simulink model "PreBrakingModel"  (Simulink 8.0)
settings: Solver=ode5  SolverMode=SingleTasking  StartTime=0.0  StopTime=inf  FixedStep=1/1000  RelTol=1e-3
libraries: simulink x27, simulink_extras x2
(part 1 of 2)
settings Model: Creator=Krzysztof  LastModifiedBy=battags  BufferReuse=off
settings DataIOCC: SignalLoggingSaveFormat=ModelDataLogs  SaveOutput=off  SaveTime=off
settings OptimizationCC: InlineParams=on  OptimizeBlockIOStorage=off  BufferReuse=off  ExpressionFolding=off  LocalBlockOutputs=off
settings DebuggingCC: SolverPrmCheckMsg=none  SigSpecEnsureSampleTimeMsg=none  ParameterPrecisionLossMsg=none  FcnCallInpInsideContextMsg=UseLocalSettings
settings ModelReferenceCC: ModelReferenceNumInstancesAllowed=Single
settings SFSimCC: SimParseCustomCode=off
settings GRTTargetCC: CombineOutputUpdateFcns=off  GRTInterface=on

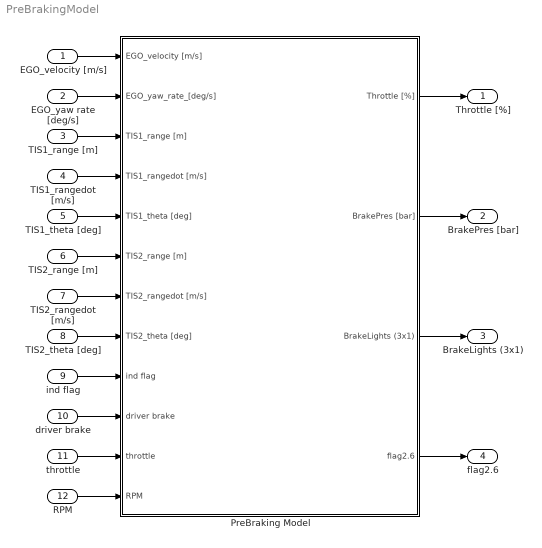
== system PreBrakingModel ==
  EGO_velocity [m/s] : Inport
  EGO_yaw rate [deg/s] : Inport  Port=2
  TIS1_range [m] : Inport  Port=3
  TIS1_rangedot [m/s] : Inport  Port=4
  TIS1_theta [deg] : Inport  Port=5
  TIS2_range [m] : Inport  Port=6
  TIS2_rangedot [m/s] : Inport  Port=7
  TIS2_theta [deg] : Inport  Port=8
  ind flag : Inport  Port=9
  driver brake : Inport  Port=10
  throttle : Inport  Port=11
  RPM : Inport  Port=12
  PreBraking Model : Subsystem  mask(PreBraking Model){MaxBrakePressure=150, BrakingPercent=0.4, LaneWidth=3.5, TISMaxRange=[150 30], TISMaxTheta=[9 80], Tblock=1/1000, Tsensor=[1/20 1/20], TISdet=[32 32], DisplaySwitch=off, DisplayFreq=20, RadarSwitch=off, RadarFreq=20}
      mask prompts: MaxBrakePressure "Maximum value of braking pressure [bar]"; BrakingPercent "Part of maximum braking pressure to use when partial braking [-]"; LaneWidth "Lane width [m]"; TISMaxRange "TIS maximum range (TIS1 and TIS2) [m]"; TISMaxTheta "TIS maximum theta angle (TIS1 and TIS2) [deg]"; Tblock "Target update rate of the compilation sheet [s]"; Tsensor "TIS update rate (TIS1 and TIS2) [s]"; TISdet "TIS max. objects to detect (TIS1 and TIS 2) [-]"; DisplaySwitch "Show EGO parameters visualization"; DisplayFreq "EGO parameters visualization frequency [Hz]"; RadarSwitch "Show radar visualization"; RadarFreq "Radar frequency [Hz]"
      mask help:
      | - intended to reduce speed of predicted collision,
      | - warns the driver and gives him more time to react,
      | - uses information from the state block
      |   and two independent TIS sensors,
      | - the system outputs are:
      |  = throttle and brake pressure (dynamics),
      |  = brake lights flags (light source visualisation animation)
      |  = the value of the warning flag.
      mask Callback DisplaySwitch:
      | en = get_param(gcb,'MaskEnables');
      | switch get_param(gcb, 'DisplaySwitch')
      |     case 'off'
      |         en{10} = 'off';
      |     case 'on'
      |         en{10} = 'on';
      | end
      | set_param(gcb,'MaskEnables',en);
      mask Callback RadarSwitch:
      | en = get_param(gcb,'MaskEnables');
      | switch get_param(gcb, 'RadarSwitch')
      |     case 'off'
      |         en{12} = 'off';
      |     case 'on'
      |         en{12} = 'on';
      | end
      | set_param(gcb,'MaskEnables',en);
  Throttle [%] : Outport
  BrakePres [bar] : Outport  Port=2
  BrakeLights (3x1) : Outport  Port=3
  flag2.6 : Outport  Port=4
  wires:
  PreBraking Model/1(Throttle [%]) -> Throttle [%]/1
  PreBraking Model/2(BrakePres [bar]) -> BrakePres [bar]/1
  PreBraking Model/3(BrakeLights (3x1)) -> BrakeLights (3x1)/1
  PreBraking Model/4(flag2.6) -> flag2.6/1
  EGO_velocity [m/s]/1 -> PreBraking Model/1(EGO_velocity [m/s])
  TIS1_range [m]/1 -> PreBraking Model/3(TIS1_range [m])
  TIS1_rangedot [m/s]/1 -> PreBraking Model/4(TIS1_rangedot [m/s])
  TIS1_theta [deg]/1 -> PreBraking Model/5(TIS1_theta [deg])
  TIS2_range [m]/1 -> PreBraking Model/6(TIS2_range [m])
  TIS2_rangedot [m/s]/1 -> PreBraking Model/7(TIS2_rangedot [m/s])
  TIS2_theta [deg]/1 -> PreBraking Model/8(TIS2_theta [deg])
  ind flag/1 -> PreBraking Model/9(ind flag)
  driver brake/1 -> PreBraking Model/10(driver brake)
  throttle/1 -> PreBraking Model/11(throttle)
  EGO_yaw rate [deg/s]/1 -> PreBraking Model/2(EGO_yaw_rate_[deg/s])
  RPM/1 -> PreBraking Model/12(RPM)

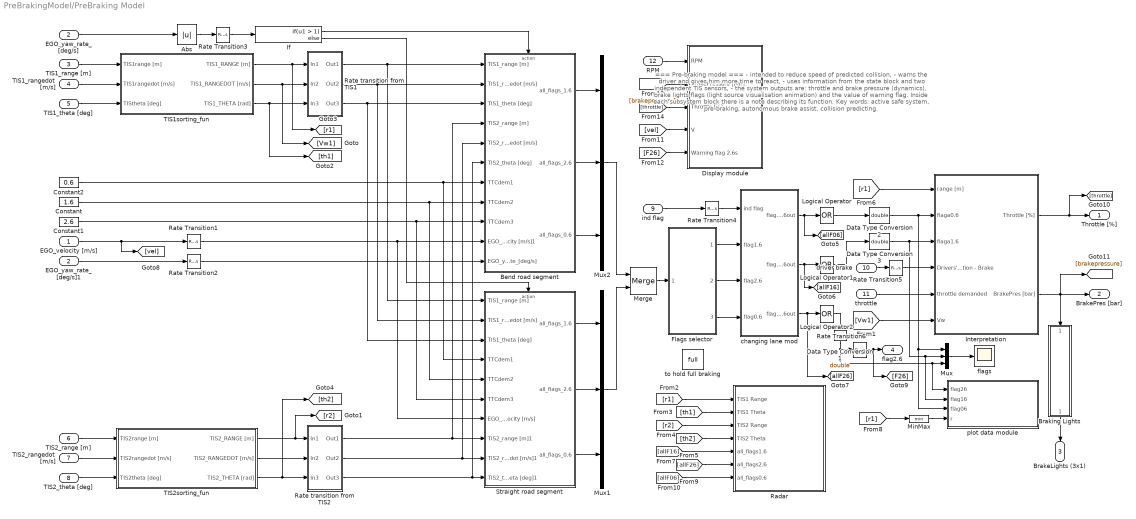
== system PreBrakingModel/PreBraking Model ==
  note: === Pre-braking model ===
      |
      |    - intended to reduce speed of predicted collision,
      |    - warns the driver and gives him more time to react,
      |    - uses information from the state block and two independent TIS sensors,
      |    - the system outputs are: throttle and brake pressure (dynamics),
      |      brake lights flags (light source visualisation animation) and the value of warning flag.
      |
      |    Inside each subsystem block there is a note describing its function.
      |
      |    Key words:
      |       active safe system, pre-braking, autonomous brake assist, collision predicting.
  EGO_velocity [m/s] : Inport  SampleTime=Tblock
  EGO_yaw_rate_[deg/s] : Inport  Port=2  SampleTime=Tblock
  TIS1_range [m] : Inport  Port=3  PortDimensions=TISdet(1)  SampleTime=Tsensor(1)
  TIS1_rangedot [m/s] : Inport  Port=4  PortDimensions=TISdet(1)  SampleTime=Tsensor(1)
  TIS1_theta [deg] : Inport  Port=5  PortDimensions=TISdet(1)  SampleTime=Tsensor(1)
  TIS2_range [m] : Inport  Port=6  PortDimensions=TISdet(2)  SampleTime=Tsensor(2)
  TIS2_rangedot [m/s] : Inport  Port=7  PortDimensions=TISdet(2)  SampleTime=Tsensor(2)
  TIS2_theta [deg] : Inport  Port=8  PortDimensions=TISdet(2)  SampleTime=Tsensor(2)
  ind flag : Inport  Port=9  SampleTime=[0 0]
  driver brake : Inport  Port=10  SampleTime=[0 0]
  throttle : Inport  Port=11  SampleTime=[0 0]
  RPM : Inport  Port=12  SampleTime=Tblock
  Abs : Abs
  Bend road segment : Subsystem  TreatAsAtomicUnit=on
  Braking Lights : Subsystem
  Constant : Constant  Value=1.6
  Constant1 : Constant  Value=2.6
  Constant2 : Constant  Value=0.6
  Data Type Conversion1 : DataTypeConversion  OutDataTypeStr=double
  Data Type Conversion2 : DataTypeConversion  OutDataTypeStr=double
  Data Type Conversion3 : DataTypeConversion  OutDataTypeStr=double
  Display module : Subsystem
  EGO_yaw_rate_[deg/s]1 : InportShadow  Port=2  SampleTime=Tblock
  Flags selector : Subsystem
  If : If  IfExpression=u1 > 1  SampleTime=min(Tsensor)
  Interpretation : Subsystem
  Logical Operator : Logic  Operator=OR  Inputs=1  AllPortsSameDT=off  OutDataTypeStr=boolean
  Logical Operator1 : Logic  Operator=OR  Inputs=1  AllPortsSameDT=off  OutDataTypeStr=boolean
  Logical Operator2 : Logic  Operator=OR  Inputs=1  AllPortsSameDT=off  OutDataTypeStr=boolean
  Merge : Merge
  MinMax : MinMax
  Mux : Mux  Inputs=3
  Mux1 : Mux  Inputs=3
  Mux2 : Mux  Inputs=3
  Radar : Subsystem
  Rate Transition{1..5} (5 alike) : RateTransition  Integrity=off  OutPortSampleTime=min(Tsensor)
  Rate Transition6 : RateTransition  Integrity=off  OutPortSampleTime=0
  Rate transition from TIS1 : Subsystem
  Rate transition from TIS2 : Subsystem
  Straight road segment : Subsystem  TreatAsAtomicUnit=on
  TIS1sorting_fun : Subsystem
  TIS2sorting_fun : Subsystem
  changing lane mod : Subsystem
  flags : Scope
      settings: TimeRange=0.1284900331530992  YMin=0.9893455251653903  YMax=1  SaveName=ScopeData26
  plot data module : Subsystem
  to hold full braking : DataStoreMemory  DataStoreName=full
  Throttle [%] : Outport
  BrakePres [bar] : Outport  Port=2
  BrakeLights (3x1) : Outport  Port=3
  flag2.6 : Outport  Port=4
  wires:
  Braking Lights/1(BrakeLights (3x1)) -> BrakeLights (3x1)/1
  driver brake/1 -> Rate Transition5/1
  throttle/1 -> Interpretation/5(throttle demanded)
  ind flag/1 -> Rate Transition4/1
  MinMax/1 -> plot data module/4(r)
  Mux/1 -> flags/1
  [r1] -> Interpretation/1(range [m])
  [r1] -> MinMax/1
  changing lane mod/1(flag0.6out) -> Logical Operator/1, [allF06]
  changing lane mod/2(flag1.6out) -> Logical Operator1/1, [allF16]
  changing lane mod/3(flag2.6out) -> Logical Operator2/1, [allF26]
  Interpretation/1(Throttle [%]) -> Throttle [%]/1, [throttle]
  If/2 -> Straight road segment/Action
  If/1 -> Bend road segment/Action
  Interpretation/2(BrakePres [bar]) -> Braking Lights/1(BrakePres), BrakePres [bar]/1, [brakepressure]
  Abs/1 -> Rate Transition3/1
  [Vw1] -> Interpretation/6(Vw)
  TIS1sorting_fun/1(TIS1_RANGE [m]) -> Rate transition from TIS1/1(In1), [r1]
  TIS1sorting_fun/2(TIS1_RANGEDOT [m/s]) -> [Vw1], Rate transition from TIS1/2(In2)
  Constant2/1 -> Bend road segment/7(TTCdem1), Straight road segment/4(TTCdem1)
  Constant/1 -> Bend road segment/8(TTCdem2), Straight road segment/5(TTCdem2)
  Constant1/1 -> Bend road segment/9(TTCdem3), Straight road segment/6(TTCdem3)
  EGO_velocity [m/s]/1 -> Rate Transition1/1, [vel]
  Mux2/1 -> Merge/1
  Mux1/1 -> Merge/2
  EGO_yaw_rate_[deg/s]1/1 -> Rate Transition2/1
  EGO_yaw_rate_[deg/s]/1 -> Abs/1
  TIS1_range [m]/1 -> TIS1sorting_fun/1(TIS1range [m])
  TIS1_rangedot [m/s]/1 -> TIS1sorting_fun/2(TIS1rangedot [m/s])
  TIS1_theta [deg]/1 -> TIS1sorting_fun/3(TIStheta [deg])
  TIS2_range [m]/1 -> TIS2sorting_fun/1(TIS2range [m])
  TIS2_rangedot [m/s]/1 -> TIS2sorting_fun/2(TIS2rangedot [m/s])
  TIS2_theta [deg]/1 -> TIS2sorting_fun/3(TIS2theta [deg])
  TIS1sorting_fun/3(TIS1_THETA [rad]) -> Rate transition from TIS1/3(In3), [th1]
  Rate transition from TIS1/1(Out1) -> Straight road segment/1(TIS1_range [m]), Bend road segment/1(TIS1_range [m])
  Rate transition from TIS1/2(Out2) -> Bend road segment/2(TIS1_rangedot [m/s]), Straight road segment/2(TIS1_rangedot [m/s])
  Rate transition from TIS1/3(Out3) -> Straight road segment/3(TIS1_theta [deg]), Bend road segment/3(TIS1_theta [deg])
  TIS2sorting_fun/1(TIS2_RANGE [m]) -> Rate transition from TIS2/1(In1), [r2]
  TIS2sorting_fun/2(TIS2_RANGEDOT [m/s]) -> Rate transition from TIS2/2(In2)
  TIS2sorting_fun/3(TIS2_THETA [rad]) -> Rate transition from TIS2/3(In3), [th2]
  Rate transition from TIS2/1(Out1) -> Straight road segment/8(TIS2_range [m]1), Bend road segment/4(TIS2_range [m])
  Rate transition from TIS2/2(Out2) -> Straight road segment/9(TIS2_rangedot [m/s]1), Bend road segment/5(TIS2_rangedot [m/s])
  Rate transition from TIS2/3(Out3) -> Straight road segment/10(TIS2_theta [deg]1), Bend road segment/6(TIS2_theta [deg])
  Rate Transition1/1 -> Bend road segment/10(EGO_velocity [m/s]1), Straight road segment/7(EGO_velocity [m/s])
  Rate Transition2/1 -> Bend road segment/11(EGO_yaw_rate_[deg/s])
  Rate Transition4/1 -> changing lane mod/1(ind flag)
  Rate Transition3/1 -> If/1
  Rate Transition5/1 -> Interpretation/4(Drivers's Reaction - Brake)
  Rate Transition6/1 -> flag2.6/1, [F26]
  Bend road segment/1(all_flags_1.6) -> Mux2/1
  Bend road segment/2(all_flags_2.6) -> Mux2/2
  Bend road segment/3(all_flags_0.6) -> Mux2/3
  Straight road segment/1(all_flags_1.6) -> Mux1/1
  Straight road segment/2(all_flags_2.6) -> Mux1/2
  Straight road segment/3(all_flags_0.6) -> Mux1/3
  Merge/1 -> Flags selector/1(all_flags)
  [r1] -> Radar/1(TIS1 Range)
  [th1] -> Radar/2(TIS1 Theta)
  [r2] -> Radar/3(TIS2 Range)
  [th2] -> Radar/4(TIS2 Theta)
  [allF16] -> Radar/5(all_flags1.6)
  [allF26] -> Radar/6(all_flags2.6)
  [allF06] -> Radar/7(all_flags0.6)
  [vel] -> Display module/4(V)
  [F26] -> Display module/5(Warning flag 2.6s)
  RPM/1 -> Display module/1(RPM)
  [brakepressure] -> Display module/2(BrakePressure [bar])
  [throttle] -> Display module/3(Throttle [%])
  Flags selector/1(all_flags1.6) -> changing lane mod/2(flag1.6)
  Flags selector/2(all_flags2.6) -> changing lane mod/3(flag2.6)
  Flags selector/3(all_flags0.6) -> changing lane mod/4(flag0.6)
  Logical Operator/1 -> Data Type Conversion2/1
  Logical Operator1/1 -> Data Type Conversion3/1
  Logical Operator2/1 -> Data Type Conversion1/1
  Data Type Conversion1/1 -> Mux/3, plot data module/1(flag26), Rate Transition6/1
  Data Type Conversion2/1 -> Mux/1, plot data module/3(flag06), Interpretation/2(flaga0.6)
  Data Type Conversion3/1 -> Interpretation/3(flaga1.6), Mux/2, plot data module/2(flag16)

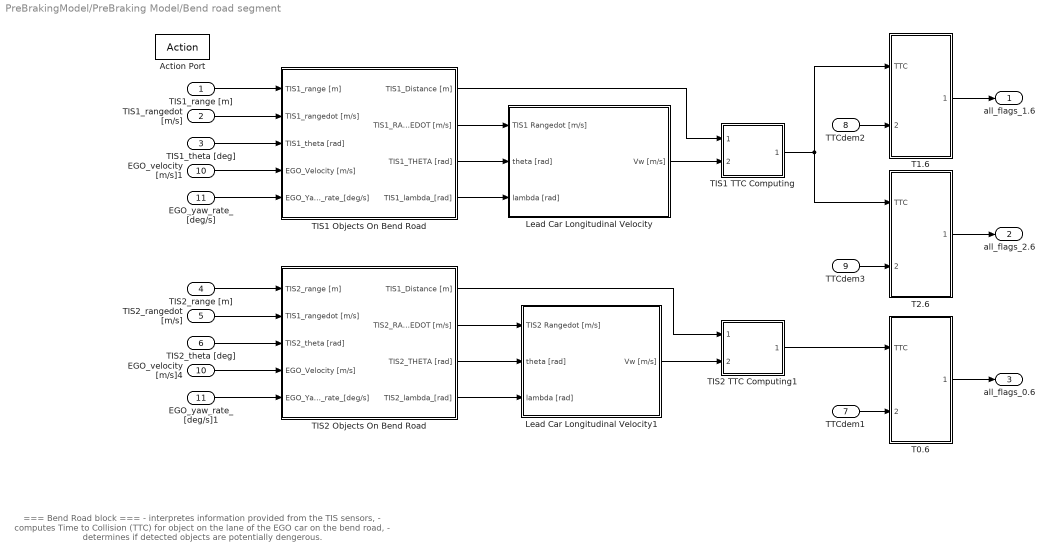
== system PreBrakingModel/PreBraking Model/Bend road segment ==
  note: === Bend Road block ===
      |
      |  - interpretes information provided from the TIS sensors,
      |  - computes Time to Collision (TTC) for object on the lane of the EGO car on the bend road,
      |  - determines if detected objects are potentially dengerous.
  TIS1_range [m] : Inport  PortDimensions=TISdet(1)
  TIS1_rangedot [m/s] : Inport  Port=2  PortDimensions=TISdet(1)
  TIS1_theta [deg] : Inport  Port=3  PortDimensions=TISdet(1)
  TIS2_range [m] : Inport  Port=4  PortDimensions=TISdet(2)
  TIS2_rangedot [m/s] : Inport  Port=5  PortDimensions=TISdet(2)
  TIS2_theta [deg] : Inport  Port=6  PortDimensions=TISdet(2)
  TTCdem1 : Inport  Port=7
  TTCdem2 : Inport  Port=8
  TTCdem3 : Inport  Port=9
  EGO_velocity [m/s]1 : Inport  Port=10
  EGO_yaw_rate_[deg/s] : Inport  Port=11
  Action Port : ActionPort  PropagateVarSize=During execution  ActionType=then
  EGO_velocity [m/s]4 : InportShadow  Port=10
  EGO_yaw_rate_[deg/s]1 : InportShadow  Port=11
  Lead Car Longitudinal Velocity : Subsystem
  Lead Car Longitudinal Velocity1 : Subsystem
  T0.6 : Subsystem
  T1.6 : Subsystem
  T2.6 : Subsystem
  TIS1 Objects On Bend Road : Subsystem
  TIS1 TTC Computing : Subsystem
  TIS2 Objects On Bend Road : Subsystem
  TIS2 TTC Computing1 : Subsystem
  all_flags_1.6 : Outport
  all_flags_2.6 : Outport  Port=2
  all_flags_0.6 : Outport  Port=3
  wires:
  EGO_yaw_rate_[deg/s]/1 -> TIS1 Objects On Bend Road/5(EGO_Yaw_rate_[deg/s])
  EGO_yaw_rate_[deg/s]1/1 -> TIS2 Objects On Bend Road/5(EGO_Yaw_rate_[deg/s])
  Lead Car Longitudinal Velocity1/1(Vw [m/s]) -> TIS2 TTC Computing1/2(Velocity [m/s])
  EGO_velocity [m/s]1/1 -> TIS1 Objects On Bend Road/4(EGO_Velocity [m/s])
  EGO_velocity [m/s]4/1 -> TIS2 Objects On Bend Road/4(EGO_Velocity [m/s])
  TIS1 Objects On Bend Road/2(TIS1_RANGEDOT [m/s]) -> Lead Car Longitudinal Velocity/1(TIS1 Rangedot [m/s])
  TIS1 Objects On Bend Road/3(TIS1_THETA [rad]) -> Lead Car Longitudinal Velocity/2(theta [rad])
  TIS1 Objects On Bend Road/4(TIS1_lambda_[rad]) -> Lead Car Longitudinal Velocity/3(lambda [rad])
  TIS2 Objects On Bend Road/1(TIS1_Distance [m]) -> TIS2 TTC Computing1/1(Distance [m])
  TIS2 Objects On Bend Road/2(TIS2_RANGEDOT [m/s]) -> Lead Car Longitudinal Velocity1/1(TIS2 Rangedot [m/s])
  TIS2 Objects On Bend Road/3(TIS2_THETA [rad]) -> Lead Car Longitudinal Velocity1/2(theta [rad])
  TIS2 Objects On Bend Road/4(TIS2_lambda_[rad]) -> Lead Car Longitudinal Velocity1/3(lambda [rad])
  TIS1 Objects On Bend Road/1(TIS1_Distance [m]) -> TIS1 TTC Computing/1(Distance [m])
  Lead Car Longitudinal Velocity/1(Vw [m/s]) -> TIS1 TTC Computing/2(Velocity [m/s])
  TIS1_range [m]/1 -> TIS1 Objects On Bend Road/1(TIS1_range [m])
  TIS1_rangedot [m/s]/1 -> TIS1 Objects On Bend Road/2(TIS1_rangedot [m/s])
  TIS1_theta [deg]/1 -> TIS1 Objects On Bend Road/3(TIS1_theta [rad])
  TIS2_range [m]/1 -> TIS2 Objects On Bend Road/1(TIS2_range [m])
  TIS2_rangedot [m/s]/1 -> TIS2 Objects On Bend Road/2(TIS1_rangedot [m/s])
  TIS2_theta [deg]/1 -> TIS2 Objects On Bend Road/3(TIS2_theta [rad])
  TTCdem2/1 -> T1.6/2(Constant TTC)
  TIS1 TTC Computing/1(TTC [s]) -> T1.6/1(TTC), T2.6/1(TTC)
  TTCdem3/1 -> T2.6/2(Constant TTC)
  TIS2 TTC Computing1/1(TTC [s]) -> T0.6/1(TTC)
  TTCdem1/1 -> T0.6/2(Constant TTC)
  T1.6/1(all_flags_1.6) -> all_flags_1.6/1
  T2.6/1(all_flags_2.6) -> all_flags_2.6/1
  T0.6/1(all_flags_0.6) -> all_flags_0.6/1

== system PreBrakingModel/PreBraking Model/Braking Lights ==
  note: === Braking lights block ===
      |
      |    - according to brake pressure, lights up braking lights of the actor,
      |    - the signal is a 3x1 vector:
      |      = first        value - left braking light,
      |      = second value - middle braking light,
      |      = third       value - right braking light.
  BrakePres : Inport
  Compare : simulink/Logic and Bit Operations/Compare To Constant  relop===  const=MaxBrakePressure  OutDataTypeStr=uint8
  Constant : Constant
  Constant1 : Constant  Value=0
  If : If  ShowElse=off  SampleTime=Tblock
  If Action Subsystem : Subsystem  TreatAsAtomicUnit=on
  Mux : Mux  Inputs=3
  Pulse Generator : DiscretePulseGenerator  Period=60  PulseWidth=30  SampleTime=Tblock
  Rate Transition2 : RateTransition  OutPortSampleTime=Tblock
  Switch : Switch  Criteria=u2 ~= 0
  Switch1 : Switch  Threshold=MaxBrakePressure
  Switch2 : Switch  Threshold=MaxBrakePressure
  BrakeLights (3x1) : Outport
  wires:
  Mux/1 -> BrakeLights (3x1)/1
  BrakePres/1 -> Rate Transition2/1
  Constant/1 -> Switch/1
  Switch/1 -> Mux/2, Switch1/3, Switch2/3
  Constant1/1 -> Switch/3
  Compare/1 -> If/1
  If/1 -> If Action Subsystem/Action
  Pulse Generator/1 -> If Action Subsystem/1(In1)
  If Action Subsystem/1(left light) -> Switch2/1
  If Action Subsystem/2(right light) -> Switch1/1
  Switch2/1 -> Mux/1
  Switch1/1 -> Mux/3
  Rate Transition2/1 -> Compare/1, Switch/2, Switch1/2, Switch2/2

== system PreBrakingModel/PreBraking Model/Display module ==
  RPM : Inport
  BrakePressure [bar] : Inport  Port=2
  Throttle [%] : Inport  Port=3
  V : Inport  Port=4
  Warning flag 2.6s : Inport  Port=5
  Display : Subsystem
  Display switch : Constant  Value=DisplaySwitch  SampleTime=1/DisplayFreq
  Gain : Gain  Gain=3.6
  Rate Transition{,1..4} (5 alike) : RateTransition  Integrity=off  OutPortSampleTime=1/DisplayFreq
  wires:
  BrakePressure [bar]/1 -> Rate Transition3/1
  Throttle [%]/1 -> Rate Transition4/1
  Warning flag 2.6s/1 -> Rate Transition/1
  RPM/1 -> Rate Transition1/1
  V/1 -> Gain/1
  Rate Transition1/1 -> Display/1(RPM)
  Rate Transition2/1 -> Display/2(V)
  Rate Transition3/1 -> Display/3(BrakePressure)
  Rate Transition4/1 -> Display/4(Throttle)
  Rate Transition/1 -> Display/5(Warning flag 2.6s)
  Display switch/1 -> Display/Enable
  Gain/1 -> Rate Transition2/1

== system PreBrakingModel/PreBraking Model/Flags selector ==
  all_flags : Inport
  Constant : Constant  Value=0
  Constant1 : Constant
  Data Store Read1 : DataStoreRead  DataStoreName=full  SampleTime=min(Tsensor)
  Data Type Conversion : DataTypeConversion
  Gain : Gain  Gain=ones(TISdet(1),1)
  Gain1 : Gain  Gain=ones(TISdet(1),1)
  Logical Operator : Logic  Operator=OR  Inputs=1  AllPortsSameDT=off  OutDataTypeStr=boolean
  Selector : Selector  InputPortWidth=2*TISdet(1)+TISdet(2)  IndexOptions=Starting index (dialog)  Indices=1  OutputSizes=TISdet(1)
  Selector1 : Selector  InputPortWidth=2*TISdet(1)+TISdet(2)  IndexOptions=Starting index (dialog)  Indices=TISdet(1)+1  OutputSizes=TISdet(1)
  Selector2 : Selector  InputPortWidth=2*TISdet(1)+TISdet(2)  IndexOptions=Starting index (dialog)  Indices=2* TISdet(1)+1  OutputSizes=TISdet(2)
  Sum : Sum  Inputs=++++
  Switch1 : Switch  Criteria=u2 > Threshold
  all_flags1.6 : Outport
  all_flags2.6 : Outport  Port=2
  all_flags0.6 : Outport  Port=3
  wires:
  Selector/1 -> all_flags1.6/1, Sum/1
  Selector2/1 -> all_flags0.6/1, Logical Operator/1
  all_flags/1 -> Data Type Conversion/1
  Data Type Conversion/1 -> Selector1/1, Selector/1, Selector2/1
  Selector1/1 -> Sum/2
  Data Store Read1/1 -> Gain/1
  Gain/1 -> Sum/4
  Logical Operator/1 -> Gain1/1
  Gain1/1 -> Sum/3
  Sum/1 -> Switch1/2
  Constant1/1 -> Switch1/1
  Constant/1 -> Switch1/3
  Switch1/1 -> all_flags2.6/1

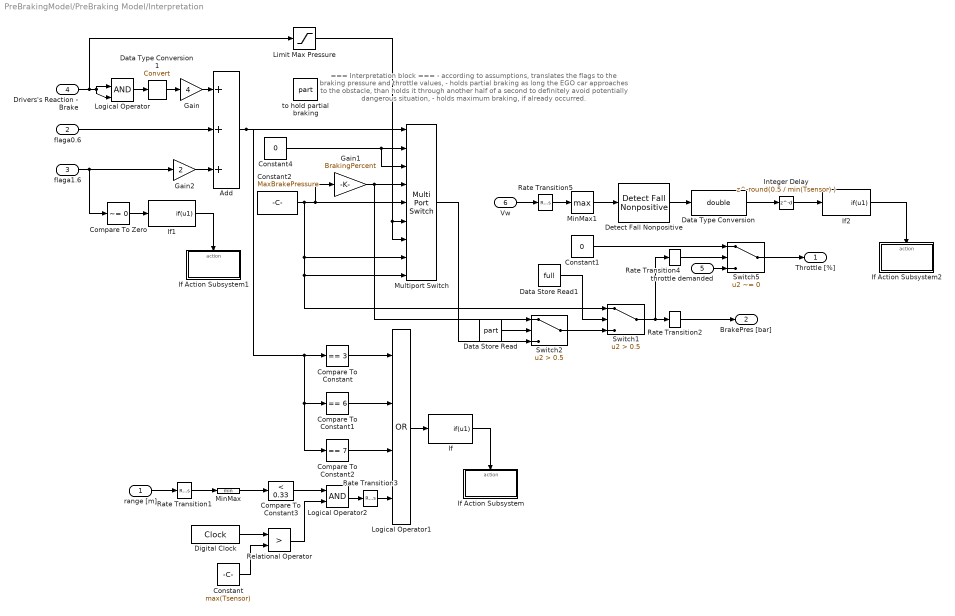
== system PreBrakingModel/PreBraking Model/Interpretation ==
  note: === Interpretation block ===
      |
      |    - according to assumptions, translates the flags
      |      to the braking pressure and throttle values,
      |    - holds partial braking as long the EGO car
      |      approaches to the obstacle, than holds it
      |      through another half of a second to definitely
      |      avoid potentially dangerous situation,
      |    - holds maximum braking, if already occurred.
  range [m] : Inport
  flaga0.6 : Inport  Port=2
  flaga1.6 : Inport  Port=3
  Drivers's Reaction - Brake : Inport  Port=4
  throttle demanded : Inport  Port=5  SampleTime=0
  Vw : Inport  Port=6
  Add : Sum  Inputs=3  SampleTime=min(Tsensor)
  Compare To Constant : simulink/Logic and Bit Operations/Compare To Constant  relop===  const=3  OutDataTypeStr=uint8
  Compare To Constant1 : simulink/Logic and Bit Operations/Compare To Constant  relop===  const=6  OutDataTypeStr=uint8
  Compare To Constant2 : simulink/Logic and Bit Operations/Compare To Constant  relop===  const=7  OutDataTypeStr=uint8
  Compare To Constant3 : simulink/Logic and Bit Operations/Compare To Constant  relop=<  const=0.33  OutDataTypeStr=uint8
  Compare To Zero : simulink/Logic and Bit Operations/Compare To Zero  relop=~=  OutDataTypeStr=uint8
  Constant : Constant  Value=max(Tsensor)
  Constant1 : Constant  Value=0  SampleTime=0
  Constant2 : Constant  Value=MaxBrakePressure  OutDataTypeStr=double  SampleTime=min(Tsensor)
  Constant4 : Constant  Value=0  SampleTime=min(Tsensor)
  Data Store Read : DataStoreRead  DataStoreName=part  SampleTime=min(Tsensor)
  Data Store Read1 : DataStoreRead  DataStoreName=full  SampleTime=min(Tsensor)
  Data Type Conversion : DataTypeConversion  OutDataTypeStr=double
  Data Type Conversion1 : DataTypeConversion
  Detect Fall Nonpositive : simulink/Logic and Bit Operations/Detect Fall Nonpositive  vinit=0  InputProcessing=Inherited  OutDataTypeStr=uint8
  Digital Clock : DigitalClock  SampleTime=min(Tsensor)
  Gain : Gain  Gain=4  SampleTime=min(Tsensor)
  Gain1 : Gain  Gain=BrakingPercent
  Gain2 : Gain  Gain=2
  If : If  IfExpression=u1  ShowElse=off  SampleTime=min(Tsensor)
  If Action Subsystem : Subsystem  TreatAsAtomicUnit=on
  If Action Subsystem1 : Subsystem  TreatAsAtomicUnit=on
  If Action Subsystem2 : Subsystem  TreatAsAtomicUnit=on
  If1 : If  IfExpression=u1  ShowElse=off
  If2 : If  IfExpression=u1  ShowElse=off  SampleTime=min(Tsensor)
  Integer Delay : Delay  DelayLength=round(0.5 / min(Tsensor) )  InputProcessing=Inherited
  Limit Max Pressure : Saturate  UpperLimit=MaxBrakePressure  LowerLimit=0  SampleTime=min(Tsensor)
  Logical Operator : Logic  IconShape=distinctive  AllPortsSameDT=off  OutDataTypeStr=boolean  SampleTime=min(Tsensor)
  Logical Operator1 : Logic  Operator=OR  Inputs=4  AllPortsSameDT=off  OutDataTypeStr=boolean  SampleTime=min(Tsensor)
  Logical Operator2 : Logic  AllPortsSameDT=off  OutDataTypeStr=boolean
  MinMax : MinMax
  MinMax1 : MinMax  Function=max
  Multiport Switch : MultiPortSwitch  DataPortOrder=Zero-based contiguous  Inputs=8  zeroidx=on
  Rate Transition1 : RateTransition  Integrity=off  OutPortSampleTime=min(Tsensor)
  Rate Transition2 : RateTransition  Integrity=off  OutPortSampleTime=0
  Rate Transition3 : RateTransition  Integrity=off  OutPortSampleTime=min(Tsensor)
  Rate Transition4 : RateTransition  Integrity=off  OutPortSampleTime=0
  Rate Transition5 : RateTransition  Integrity=off  OutPortSampleTime=min(Tsensor)
  Relational Operator : RelationalOperator  Operator=>  OutDataTypeStr=boolean  SampleTime=min(Tsensor)
  Switch1 : Switch  Criteria=u2 > Threshold  Threshold=0.5  SampleTime=min(Tsensor)
  Switch2 : Switch  Criteria=u2 > Threshold  Threshold=0.5  SampleTime=min(Tsensor)
  Switch5 : Switch  Criteria=u2 ~= 0
  to hold partial braking : DataStoreMemory  DataStoreName=part
  Throttle [%] : Outport  SampleTime=0
  BrakePres [bar] : Outport  Port=2
  wires:
  flaga1.6/1 -> Gain2/1, Compare To Zero/1
  Drivers's Reaction - Brake/1 -> Logical Operator/1, Logical Operator/2, Limit Max Pressure/1
  Gain2/1 -> Add/3
  Add/1 -> Multiport Switch/1, Compare To Constant1/1, Compare To Constant2/1, Compare To Constant/1
  Constant2/1 -> Gain1/1, Multiport Switch/5, Multiport Switch/8, Multiport Switch/9, Switch1/1
  flaga0.6/1 -> Add/2
  Gain/1 -> Add/1
  Multiport Switch/1 -> Switch2/3
  throttle demanded/1 -> Switch5/3
  Logical Operator/1 -> Data Type Conversion1/1
  Constant4/1 -> Multiport Switch/2, Multiport Switch/3
  Gain1/1 -> Multiport Switch/4, Switch2/1
  Limit Max Pressure/1 -> Multiport Switch/6, Multiport Switch/7
  range [m]/1 -> Rate Transition1/1
  Compare To Constant/1 -> Logical Operator1/1
  Compare To Constant1/1 -> Logical Operator1/2
  Compare To Constant2/1 -> Logical Operator1/3
  Logical Operator1/1 -> If/1
  Data Store Read/1 -> Switch2/2
  If/1 -> If Action Subsystem/Action
  MinMax/1 -> Compare To Constant3/1
  If1/1 -> If Action Subsystem1/Action
  Data Store Read1/1 -> Switch1/2
  Switch2/1 -> Switch1/3
  Compare To Zero/1 -> If1/1
  Vw/1 -> Rate Transition5/1
  MinMax1/1 -> Detect Fall Nonpositive/1
  If2/1 -> If Action Subsystem2/Action
  Detect Fall Nonpositive/1 -> Data Type Conversion/1
  Data Type Conversion/1 -> Integer Delay/1
  Integer Delay/1 -> If2/1
  Switch5/1 -> Throttle [%]/1
  Switch1/1 -> Rate Transition4/1, Rate Transition2/1
  Constant1/1 -> Switch5/1
  Rate Transition1/1 -> MinMax/1
  Digital Clock/1 -> Relational Operator/1
  Logical Operator2/1 -> Rate Transition3/1
  Compare To Constant3/1 -> Logical Operator2/1
  Relational Operator/1 -> Logical Operator2/2
  Rate Transition3/1 -> Logical Operator1/4
  Constant/1 -> Relational Operator/2
  Rate Transition5/1 -> MinMax1/1
  Rate Transition4/1 -> Switch5/2
  Rate Transition2/1 -> BrakePres [bar]/1
  Data Type Conversion1/1 -> Gain/1

== system PreBrakingModel/PreBraking Model/Radar ==
  TIS1 Range : Inport
  TIS1 Theta : Inport  Port=2
  TIS2 Range : Inport  Port=3
  TIS2 Theta : Inport  Port=4
  all_flags1.6 : Inport  Port=5
  all_flags2.6 : Inport  Port=6
  all_flags0.6 : Inport  Port=7
  Radar : Subsystem
  Radar switch : Constant  Value=RadarSwitch
  Rate Transition{1..7} (7 alike) : RateTransition  Integrity=off  OutPortSampleTime=1/RadarFreq
  wires:
  TIS1 Range/1 -> Rate Transition5/1
  TIS1 Theta/1 -> Rate Transition1/1
  TIS2 Range/1 -> Rate Transition2/1
  TIS2 Theta/1 -> Rate Transition3/1
  all_flags1.6/1 -> Rate Transition4/1
  all_flags2.6/1 -> Rate Transition6/1
  all_flags0.6/1 -> Rate Transition7/1
  Rate Transition5/1 -> Radar/1(TIS1 Range)
  Rate Transition1/1 -> Radar/2(TIS1 Theta)
  Rate Transition2/1 -> Radar/3(TIS2 Range)
  Rate Transition3/1 -> Radar/4(TIS2 Theta)
  Rate Transition4/1 -> Radar/5(all_flags1.6)
  Rate Transition6/1 -> Radar/6(all_flags2.6)
  Rate Transition7/1 -> Radar/7(all_flags0.6)
  Radar switch/1 -> Radar/Enable

== system PreBrakingModel/PreBraking Model/Rate transition from TIS1 ==
  In1 : Inport
  In2 : Inport  Port=2
  In3 : Inport  Port=3
  Rate Transition1 : RateTransition  Integrity=off  OutPortSampleTime=min(Tsensor)
  Rate Transition2 : RateTransition  Integrity=off  OutPortSampleTime=min(Tsensor)
  Rate Transition3 : RateTransition  Integrity=off  OutPortSampleTime=min(Tsensor)
  Out1 : Outport
  Out2 : Outport  Port=2
  Out3 : Outport  Port=3
  wires:
  In1/1 -> Rate Transition1/1
  Rate Transition1/1 -> Out1/1
  In2/1 -> Rate Transition2/1
  Rate Transition2/1 -> Out2/1
  In3/1 -> Rate Transition3/1
  Rate Transition3/1 -> Out3/1

== system PreBrakingModel/PreBraking Model/Rate transition from TIS2 ==
  In1 : Inport
  In2 : Inport  Port=2
  In3 : Inport  Port=3
  Rate Transition1 : RateTransition  Integrity=off  OutPortSampleTime=min(Tsensor)
  Rate Transition2 : RateTransition  Integrity=off  OutPortSampleTime=min(Tsensor)
  Rate Transition3 : RateTransition  Integrity=off  OutPortSampleTime=min(Tsensor)
  Out1 : Outport
  Out2 : Outport  Port=2
  Out3 : Outport  Port=3
  wires:
  Rate Transition3/1 -> Out3/1
  In3/1 -> Rate Transition3/1
  Rate Transition2/1 -> Out2/1
  In2/1 -> Rate Transition2/1
  Rate Transition1/1 -> Out1/1
  In1/1 -> Rate Transition1/1

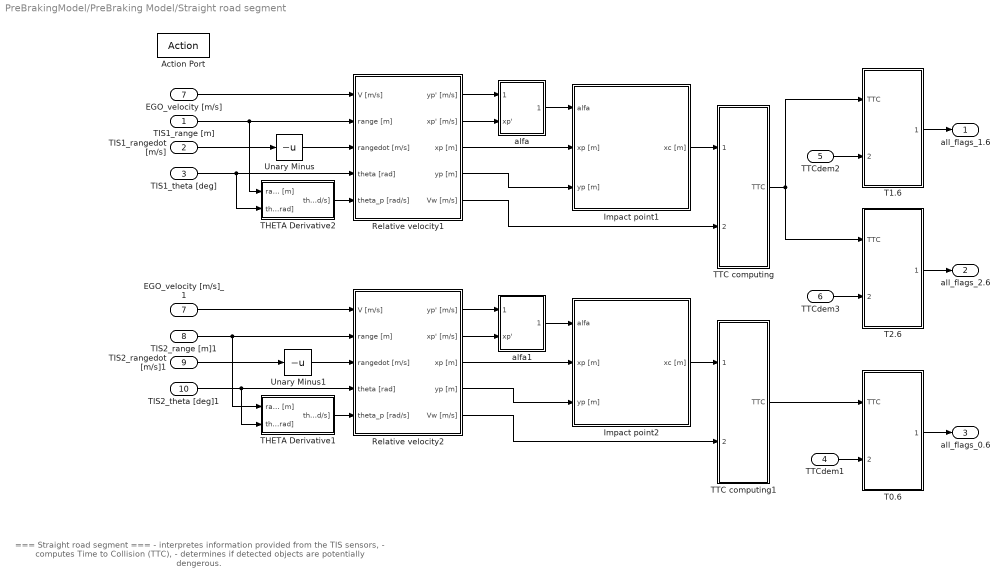
== system PreBrakingModel/PreBraking Model/Straight road segment ==
  note: === Straight road segment ===
      |
      |  - interpretes information provided from the TIS sensors,
      |  - computes Time to Collision (TTC),
      |  - determines if detected objects are potentially dengerous.
  TIS1_range [m] : Inport  PortDimensions=TISdet(1)
  TIS1_rangedot [m/s] : Inport  Port=2  PortDimensions=TISdet(1)
  TIS1_theta [deg] : Inport  Port=3  PortDimensions=TISdet(1)
  TTCdem1 : Inport  Port=4
  TTCdem2 : Inport  Port=5
  TTCdem3 : Inport  Port=6
  EGO_velocity [m/s] : Inport  Port=7
  TIS2_range [m]1 : Inport  Port=8  PortDimensions=TISdet(2)
  TIS2_rangedot [m/s]1 : Inport  Port=9  PortDimensions=TISdet(2)
  TIS2_theta [deg]1 : Inport  Port=10  PortDimensions=TISdet(2)
  Action Port : ActionPort  PropagateVarSize=During execution  ActionType=else
  EGO_velocity [m/s]_1 : InportShadow  Port=7
  Impact point1 : Subsystem
  Impact point2 : Subsystem
  Relative velocity1 : Subsystem
  Relative velocity2 : Subsystem
  T0.6 : Subsystem
  T1.6 : Subsystem
  T2.6 : Subsystem
  THETA Derivative1 : Subsystem
  THETA Derivative2 : Subsystem
  TTC computing : Subsystem
  TTC computing1 : Subsystem
  Unary Minus : UnaryMinus
  Unary Minus1 : UnaryMinus
  alfa : Subsystem
  alfa1 : Subsystem
  all_flags_1.6 : Outport
  all_flags_2.6 : Outport  Port=2
  all_flags_0.6 : Outport  Port=3
  wires:
  EGO_velocity [m/s]/1 -> Relative velocity1/1(V [m/s])
  TIS1_range [m]/1 -> Relative velocity1/2(range [m]), THETA Derivative2/1(range [m])
  TIS1_rangedot [m/s]/1 -> Unary Minus/1
  TIS1_theta [deg]/1 -> Relative velocity1/4(theta [rad]), THETA Derivative2/2(theta [rad])
  THETA Derivative2/1(theta_dot [rad/s]) -> Relative velocity1/5(theta_p [rad/s])
  Relative velocity1/1(yp' [m/s]) -> alfa/1(yp'1)
  Relative velocity1/2(xp' [m/s]) -> alfa/2(xp')
  Relative velocity1/3(xp [m]) -> Impact point1/2(xp [m])
  Relative velocity1/4(yp [m]) -> Impact point1/3(yp [m])
  EGO_velocity [m/s]_1/1 -> Relative velocity2/1(V [m/s])
  TIS2_range [m]1/1 -> THETA Derivative1/1(range [m]), Relative velocity2/2(range [m])
  TIS2_rangedot [m/s]1/1 -> Unary Minus1/1
  TIS2_theta [deg]1/1 -> Relative velocity2/4(theta [rad]), THETA Derivative1/2(theta [rad])
  THETA Derivative1/1(theta_dot [rad/s]) -> Relative velocity2/5(theta_p [rad/s])
  Relative velocity2/1(yp' [m/s]) -> alfa1/1(yp'1)
  Relative velocity2/2(xp' [m/s]) -> alfa1/2(xp')
  Relative velocity2/3(xp [m]) -> Impact point2/2(xp [m])
  alfa/1(alfa1) -> Impact point1/1(alfa)
  Impact point1/1(xc [m]) -> TTC computing/1(xc [m])
  alfa1/1(alfa1) -> Impact point2/1(alfa)
  Relative velocity1/5(Vw [m/s]) -> TTC computing/2(Vw [m/s])
  Unary Minus/1 -> Relative velocity1/3(rangedot [m/s])
  Unary Minus1/1 -> Relative velocity2/3(rangedot [m/s])
  Relative velocity2/4(yp [m]) -> Impact point2/3(yp [m])
  Impact point2/1(xc [m]) -> TTC computing1/1(xc [m])
  Relative velocity2/5(Vw [m/s]) -> TTC computing1/2(Vw [m/s])
  TTC computing/1(TTC) -> T1.6/1(TTC), T2.6/1(TTC)
  TTC computing1/1(TTC) -> T0.6/1(TTC)
  TTCdem2/1 -> T1.6/2(Constant TTC)
  TTCdem3/1 -> T2.6/2(Constant TTC)
  TTCdem1/1 -> T0.6/2(Constant TTC)
  T1.6/1(all_flags_1.6) -> all_flags_1.6/1
  T2.6/1(all_flags_2.6) -> all_flags_2.6/1
  T0.6/1(all_flags_0,6) -> all_flags_0.6/1

== system PreBrakingModel/PreBraking Model/TIS1sorting_fun ==
  note: === Sorting block ===
      |
      |    - sorts the output of the TIS sensor: range, rangedot and theta
      |      to decrease number of discontinuities of the signals values,
      |    - if nothing is detected, range value is switched from 0 to maximum,
      |    - theta signal is unary minused to switch axis system from {range, azimuth, elevation}
      |       to carthesian counter-clockwise,
      |    - cuts off signals with near-maksimum theta value.
  TIS1range [m] : Inport
  TIS1rangedot [m/s] : Inport  Port=2
  TIStheta [deg] : Inport  Port=3
  Degrees to Radians : simulink_extras/Transformations/Degrees to Radians
  Embedded MATLAB Function : MATLAB Function  TreatAsAtomicUnit=on
  Embedded MATLAB Function1 : MATLAB Function  TreatAsAtomicUnit=on
  Embedded MATLAB Function2 : MATLAB Function  TreatAsAtomicUnit=on
  MATLAB Function : MATLAB Function  TreatAsAtomicUnit=on
  Switch : Switch  Criteria=u2 ~= 0
  Unary Minus : UnaryMinus
  Unary Minus2 : UnaryMinus
  Unit Delay : UnitDelay  InitialCondition=[ 1:TISdet(1) ]  SampleTime=-1
  range max : Constant  Value=TISMaxRange(1)
  TIS1_RANGE [m] : Outport
  TIS1_RANGEDOT [m/s] : Outport  Port=2
  TIS1_THETA [rad] : Outport  Port=3
  wires:
  Unary Minus/1 -> Degrees to Radians/1
  Switch/1 -> TIS1_RANGE [m]/1
  Degrees to Radians/1 -> TIS1_THETA [rad]/1
  TIStheta [deg]/1 -> Embedded MATLAB Function1/2(theta)
  MATLAB Function/1(indx) -> Embedded MATLAB Function1/1(indx), Embedded MATLAB Function2/1(indx), Embedded MATLAB Function/2(indx), Unit Delay/1
  Unit Delay/1 -> MATLAB Function/1(indxp)
  TIS1range [m]/1 -> Embedded MATLAB Function/1(range), MATLAB Function/2(range)
  TIS1rangedot [m/s]/1 -> Embedded MATLAB Function2/2(rangedot)
  Unary Minus2/1 -> TIS1_RANGEDOT [m/s]/1
  Embedded MATLAB Function2/1(RANGEDOT) -> Unary Minus2/1
  Embedded MATLAB Function1/1(THETA) -> Unary Minus/1
  range max/1 -> Switch/3
  Embedded MATLAB Function/1(RANGE) -> Switch/2, Switch/1

== system PreBrakingModel/PreBraking Model/TIS2sorting_fun ==
  note: === Sorting block ===
      |
      |    - sorts the output of the TIS sensor: range, rangedot and theta
      |      to decrease number of discontinuities of the signals values,
      |    - uses external script,
      |    - if nothing is detected, range value is switched from 0 to maximum,
      |    - theta signal is unary minused to switch axis system from {range, azimuth, elevation}
      |       to carthesian counter-clockwise,
      |    - cuts off signals with near-maksimum theta value.
  TIS2range [m] : Inport
  TIS2rangedot [m/s] : Inport  Port=2
  TIS2theta [deg] : Inport  Port=3
  Degrees to Radians : simulink_extras/Transformations/Degrees to Radians
  Embedded MATLAB Function : MATLAB Function  TreatAsAtomicUnit=on
  Embedded MATLAB Function1 : MATLAB Function  TreatAsAtomicUnit=on
  Embedded MATLAB Function2 : MATLAB Function  TreatAsAtomicUnit=on
  MATLAB Function : MATLAB Function  TreatAsAtomicUnit=on
  Switch : Switch  Criteria=u2 ~= 0
  Unary Minus : UnaryMinus
  Unary Minus2 : UnaryMinus
  Unit Delay : UnitDelay  InitialCondition=[ 1 : TISdet(2) ]  SampleTime=-1
  range max : Constant  Value=5*TISMaxRange(2)
  TIS2_RANGE [m] : Outport
  TIS2_RANGEDOT [m/s] : Outport  Port=2
  TIS2_THETA [rad] : Outport  Port=3
  wires:
  Switch/1 -> TIS2_RANGE [m]/1
  Degrees to Radians/1 -> TIS2_THETA [rad]/1
  Unary Minus/1 -> Degrees to Radians/1
  range max/1 -> Switch/3
  MATLAB Function/1(indx) -> Embedded MATLAB Function1/1(indx), Embedded MATLAB Function2/1(indx), Embedded MATLAB Function/2(indx), Unit Delay/1
  Unit Delay/1 -> MATLAB Function/1(indxp)
  TIS2range [m]/1 -> Embedded MATLAB Function/1(range), MATLAB Function/2(range)
  TIS2rangedot [m/s]/1 -> Embedded MATLAB Function2/2(rangedot)
  Embedded MATLAB Function/1(RANGE) -> Switch/2, Switch/1
  Embedded MATLAB Function2/1(RANGEDOT) -> Unary Minus2/1
  Embedded MATLAB Function1/1(THETA) -> Unary Minus/1
  TIS2theta [deg]/1 -> Embedded MATLAB Function1/2(theta)
  Unary Minus2/1 -> TIS2_RANGEDOT [m/s]/1

== system PreBrakingModel/PreBraking Model/changing lane mod ==
  note: === Changing lane mod block ===
      |
      |    - if indicator flag is high (driver intends to turn or overtake),
      |      outputs low levels of flags, so the system will not turn on.
  ind flag : Inport
  flag1.6 : Inport  Port=2
  flag2.6 : Inport  Port=3
  flag0.6 : Inport  Port=4
  Constant : Constant  Value=0
  Data Type Conversion : DataTypeConversion  OutDataTypeStr=double
  Demux : Demux  Outputs=3
  Mux : Mux  Inputs=3
  Switch : Switch  Criteria=u2 > Threshold
  flag0.6out : Outport
  flag1.6out : Outport  Port=2
  flag2.6out : Outport  Port=3
  wires:
  flag0.6/1 -> Mux/2
  ind flag/1 -> Switch/2
  Constant/1 -> Switch/1
  Switch/1 -> Demux/1
  Mux/1 -> Data Type Conversion/1
  flag1.6/1 -> Mux/1
  flag2.6/1 -> Mux/3
  Demux/2 -> flag0.6out/1
  Demux/1 -> flag1.6out/1
  Data Type Conversion/1 -> Switch/3
  Demux/3 -> flag2.6out/1

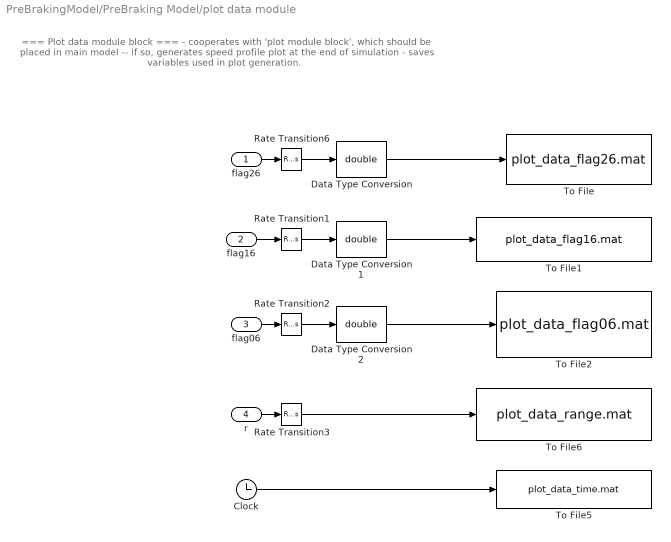
== system PreBrakingModel/PreBraking Model/plot data module ==
  note: === Plot data module block ===
      |
      |    - cooperates with 'plot module block', which should be placed in main model
      |       -- if so, generates speed profile plot at the end of simulation
      |    - saves variables used in plot generation.
  flag26 : Inport
  flag16 : Inport  Port=2
  flag06 : Inport  Port=3
  r : Inport  Port=4
  Clock : Clock
  Data Type Conversion : DataTypeConversion  OutDataTypeStr=double
  Data Type Conversion1 : DataTypeConversion  OutDataTypeStr=double
  Data Type Conversion2 : DataTypeConversion  OutDataTypeStr=double
  Rate Transition{1..3,6} (4 alike) : RateTransition  Integrity=off  OutPortSampleTime=0
  To File : ToFile  Filename=plot_data_flag26.mat  MatrixName=flag26
  To File1 : ToFile  Filename=plot_data_flag16.mat  MatrixName=flag16
  To File2 : ToFile  Filename=plot_data_flag06.mat  MatrixName=flag06
  To File5 : ToFile  Filename=plot_data_time.mat  MatrixName=time
  To File6 : ToFile  Filename=plot_data_range.mat  MatrixName=range
  wires:
  flag26/1 -> Rate Transition6/1
  flag16/1 -> Rate Transition1/1
  flag06/1 -> Rate Transition2/1
  r/1 -> Rate Transition3/1
  Data Type Conversion/1 -> To File/1
  Data Type Conversion1/1 -> To File1/1
  Data Type Conversion2/1 -> To File2/1
  Clock/1 -> To File5/1
  Rate Transition6/1 -> Data Type Conversion/1
  Rate Transition1/1 -> Data Type Conversion1/1
  Rate Transition2/1 -> Data Type Conversion2/1
  Rate Transition3/1 -> To File6/1

== system PreBrakingModel/PreBraking Model/Bend road segment/Lead Car Longitudinal Velocity ==
  note: === TIS1 Lead Car Longitudinal Velocity block ===
      |
      |  - computes relative velocity between the EGO and leading car.
  TIS1 Rangedot [m/s] : Inport
  theta [rad] : Inport  Port=2
  lambda [rad] : Inport  Port=3
  Add1 : Sum  Inputs=+-
  Constant : Constant  Value=0
  Divide2 : Product  Inputs=*/
  Switch1 : Switch  Criteria=u2 ~= 0
  TIS1 Rangedot [m/s]1 : InportShadow
  Trigonometric Function : Trigonometry  Operator=cos
  Vw [m/s] : Outport
  wires:
  TIS1 Rangedot [m/s]/1 -> Divide2/1
  lambda [rad]/1 -> Add1/1
  theta [rad]/1 -> Add1/2
  Add1/1 -> Trigonometric Function/1
  Trigonometric Function/1 -> Divide2/2
  Divide2/1 -> Switch1/1
  Switch1/1 -> Vw [m/s]/1
  TIS1 Rangedot [m/s]1/1 -> Switch1/2
  Constant/1 -> Switch1/3

== system PreBrakingModel/PreBraking Model/Bend road segment/Lead Car Longitudinal Velocity1 ==
  note: === TIS1 Lead Car Longitudinal Velocity block ===
      |
      |  - computes relative velocity between the EGO and leading car.
  TIS2 Rangedot [m/s] : Inport
  theta [rad] : Inport  Port=2
  lambda [rad] : Inport  Port=3
  Add1 : Sum  Inputs=+-
  Constant : Constant  Value=0
  Divide2 : Product  Inputs=*/
  Switch1 : Switch  Criteria=u2 ~= 0
  TIS1 Rangedot [m/s]1 : InportShadow
  Trigonometric Function : Trigonometry  Operator=cos
  Vw [m/s] : Outport
  wires:
  TIS2 Rangedot [m/s]/1 -> Divide2/1
  lambda [rad]/1 -> Add1/1
  theta [rad]/1 -> Add1/2
  Add1/1 -> Trigonometric Function/1
  Trigonometric Function/1 -> Divide2/2
  Divide2/1 -> Switch1/1
  Switch1/1 -> Vw [m/s]/1
  TIS1 Rangedot [m/s]1/1 -> Switch1/2
  Constant/1 -> Switch1/3

== system PreBrakingModel/PreBraking Model/Bend road segment/T0.6 ==
  note: === T1.6 block ==
      |
      |    - compare TTC and output adequate binary vector flag.
  TTC : Inport
  Constant TTC : Inport  Port=2
  Gain : Gain  Gain=2
  Gain1 : Gain  Gain=ones(TISdet(2),1)
  Relational Operator1 : RelationalOperator  Operator=<  OutDataTypeStr=fixdt(1,16)
  Switch : Switch  Criteria=u2 > Threshold
  all_flags_0.6 : Outport
  wires:
  Switch/1 -> Relational Operator1/1
  Relational Operator1/1 -> all_flags_0.6/1
  TTC/1 -> Switch/2, Switch/1
  Gain/1 -> Switch/3
  Constant TTC/1 -> Gain1/1
  Gain1/1 -> Gain/1, Relational Operator1/2

== system PreBrakingModel/PreBraking Model/Bend road segment/T1.6 ==
  note: === T1.6 block ==
      |
      |    - compare TTC and output adequate binary vector flag.
  TTC : Inport
  Constant TTC : Inport  Port=2
  Gain : Gain  Gain=2
  Gain1 : Gain  Gain=ones(TISdet(1),1)
  Relational Operator1 : RelationalOperator  Operator=<  OutDataTypeStr=fixdt(1,16)
  Switch : Switch  Criteria=u2 > Threshold
  median filter : Subsystem
  all_flags_1.6 : Outport
  wires:
  Switch/1 -> Relational Operator1/1
  Relational Operator1/1 -> median filter/1(Flag in)
  TTC/1 -> Switch/2, Switch/1
  Gain/1 -> Switch/3
  Constant TTC/1 -> Gain1/1
  Gain1/1 -> Gain/1, Relational Operator1/2
  median filter/1(Flag out) -> all_flags_1.6/1

== system PreBrakingModel/PreBraking Model/Bend road segment/T2.6 ==
  note: === T1.6 block ==
      |
      |    - compare TTC and output adequate binary vector flag.
  TTC : Inport
  Constant TTC : Inport  Port=2
  Gain : Gain  Gain=2
  Gain1 : Gain  Gain=ones(TISdet(1),1)
  Relational Operator1 : RelationalOperator  Operator=<  OutDataTypeStr=fixdt(1,16)
  Switch : Switch  Criteria=u2 > Threshold
  median filter : Subsystem
  all_flags_2.6 : Outport
  wires:
  Switch/1 -> Relational Operator1/1
  Relational Operator1/1 -> median filter/1(Flag in)
  TTC/1 -> Switch/2, Switch/1
  Gain/1 -> Switch/3
  Constant TTC/1 -> Gain1/1
  Gain1/1 -> Gain/1, Relational Operator1/2
  median filter/1(Flag out) -> all_flags_2.6/1

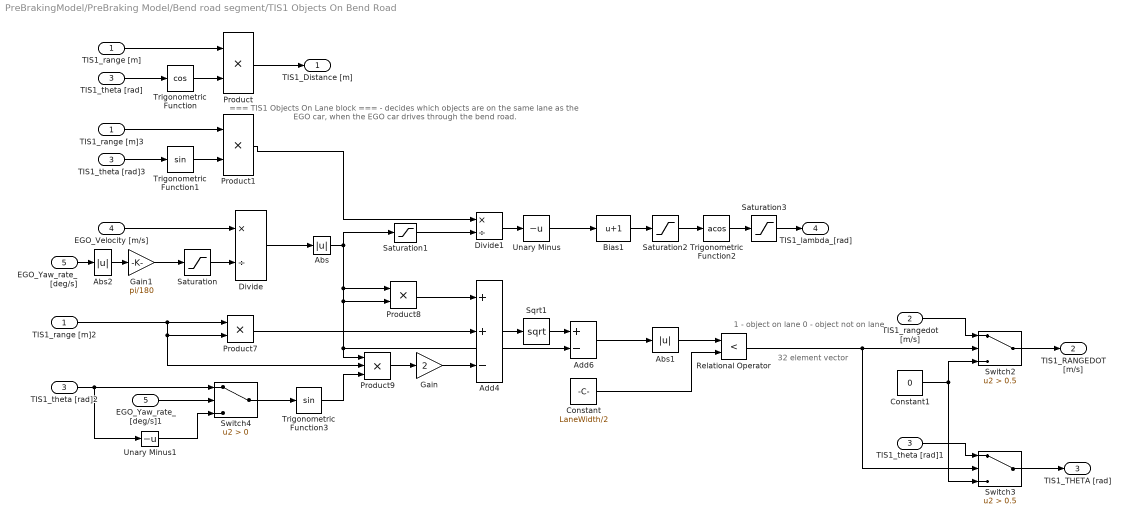
== system PreBrakingModel/PreBraking Model/Bend road segment/TIS1 Objects On Bend Road ==
  note: 1  - object      on lane
      | 0 - object not on lane
  note: 32 element vector
  note: === TIS1 Objects On Lane block ===
      |
      |  - decides which objects are on the same lane as the EGO car,
      |     when the EGO car drives through the bend road.
  TIS1_range [m] : Inport
  TIS1_rangedot [m/s] : Inport  Port=2
  TIS1_theta [rad] : Inport  Port=3
  EGO_Velocity [m/s] : Inport  Port=4
  EGO_Yaw_rate_[deg/s] : Inport  Port=5
  Abs : Abs
  Abs1 : Abs
  Abs2 : Abs
  Add4 : Sum  Inputs=++-
  Add6 : Sum  Inputs=+-
  Bias1 : Bias  Bias=1
  Constant : Constant  Value=LaneWidth/2
  Constant1 : Constant  Value=0
  Divide : Product  Inputs=*/
  Divide1 : Product  Inputs=*/
  EGO_Yaw_rate_[deg/s]1 : InportShadow  Port=5
  Gain : Gain  Gain=2
  Gain1 : Gain  Gain=pi/180
  Product{,1,7..8} (4 alike) : Product  RndMeth=Zero
  Product9 : Product  Inputs=3  RndMeth=Zero
  Relational Operator : RelationalOperator  Operator=<  OutDataTypeStr=boolean
  Saturation : Saturate  UpperLimit=inf  LowerLimit=1e-6
  Saturation1 : Saturate  UpperLimit=inf  LowerLimit=1e-6
  Saturation2 : Saturate  UpperLimit=1  LowerLimit=-1
  Saturation3 : Saturate  UpperLimit=pi  LowerLimit=0
  Sqrt1 : Math  Operator=sqrt  SaturateOnIntegerOverflow=on
  Switch2 : Switch  Criteria=u2 > Threshold  Threshold=0.5
  Switch3 : Switch  Criteria=u2 > Threshold  Threshold=0.5
  Switch4 : Switch  Criteria=u2 > Threshold
  TIS1_range [m]2 : InportShadow
  TIS1_range [m]3 : InportShadow
  TIS1_theta [rad]1 : InportShadow  Port=3
  TIS1_theta [rad]2 : InportShadow  Port=3
  TIS1_theta [rad]3 : InportShadow  Port=3
  Trigonometric Function : Trigonometry  Operator=cos
  Trigonometric Function1 : Trigonometry
  Trigonometric Function2 : Trigonometry  Operator=acos
  Trigonometric Function3 : Trigonometry
  Unary Minus : UnaryMinus
  Unary Minus1 : UnaryMinus
  TIS1_Distance [m] : Outport
  TIS1_RANGEDOT [m/s] : Outport  Port=2
  TIS1_THETA [rad] : Outport  Port=3
  TIS1_lambda_[rad] : Outport  Port=4
  wires:
  TIS1_range [m]/1 -> Product/1
  TIS1_theta [rad]/1 -> Trigonometric Function/1
  Trigonometric Function/1 -> Product/2
  Trigonometric Function1/1 -> Product1/2
  EGO_Velocity [m/s]/1 -> Divide/1
  EGO_Yaw_rate_[deg/s]/1 -> Abs2/1
  Divide/1 -> Abs/1
  Relational Operator/1 -> Switch2/2, Switch3/2
  TIS1_rangedot [m/s]/1 -> Switch2/1
  TIS1_theta [rad]1/1 -> Switch3/1
  Constant1/1 -> Switch2/3, Switch3/3
  Switch2/1 -> TIS1_RANGEDOT [m/s]/1
  Switch3/1 -> TIS1_THETA [rad]/1
  Bias1/1 -> Saturation2/1
  Divide1/1 -> Unary Minus/1
  Unary Minus/1 -> Bias1/1
  Trigonometric Function2/1 -> Saturation3/1
  Abs/1 -> Product8/1, Product8/2, Product9/1, Add6/2, Saturation1/1
  Product/1 -> TIS1_Distance [m]/1
  Product8/1 -> Add4/1
  Product7/1 -> Add4/2
  Gain/1 -> Add4/3
  Product9/1 -> Gain/1
  Trigonometric Function3/1 -> Product9/3
  Add4/1 -> Sqrt1/1
  Sqrt1/1 -> Add6/1
  Add6/1 -> Abs1/1
  EGO_Yaw_rate_[deg/s]1/1 -> Switch4/2
  Switch4/1 -> Trigonometric Function3/1
  TIS1_theta [rad]2/1 -> Switch4/1, Unary Minus1/1
  Unary Minus1/1 -> Switch4/3
  TIS1_range [m]2/1 -> Product7/1, Product7/2, Product9/2
  TIS1_range [m]3/1 -> Product1/1
  TIS1_theta [rad]3/1 -> Trigonometric Function1/1
  Product1/1 -> Divide1/1
  Abs1/1 -> Relational Operator/1
  Constant/1 -> Relational Operator/2
  Saturation/1 -> Divide/2
  Saturation1/1 -> Divide1/2
  Saturation2/1 -> Trigonometric Function2/1
  Saturation3/1 -> TIS1_lambda_[rad]/1
  Gain1/1 -> Saturation/1
  Abs2/1 -> Gain1/1

== system PreBrakingModel/PreBraking Model/Bend road segment/TIS1 TTC Computing ==
  Distance [m] : Inport
  Velocity [m/s] : Inport  Port=2
  Compare : simulink/Logic and Bit Operations/Compare To Constant  relop===  const=1e-6  OutDataTypeStr=uint8  ZeroCross=off
  Constant : Constant  Value=0
  Data Type Conversion : DataTypeConversion
  Product : Product  Inputs=*/  RndMeth=Zero
  Saturation : Saturate  UpperLimit=inf  LowerLimit=1e-6
  Switch : Switch  Criteria=u2 > Threshold
  Switch1 : Switch  Criteria=u2 > Threshold  Threshold=0.5
  TTC [s] : Outport
  wires:
  Velocity [m/s]/1 -> Switch/2, Switch/1
  Constant/1 -> Switch/3, Switch1/1
  Switch/1 -> Saturation/1
  Distance [m]/1 -> Product/1
  Saturation/1 -> Product/2, Compare/1
  Compare/1 -> Data Type Conversion/1
  Product/1 -> Switch1/3
  Switch1/1 -> TTC [s]/1
  Data Type Conversion/1 -> Switch1/2

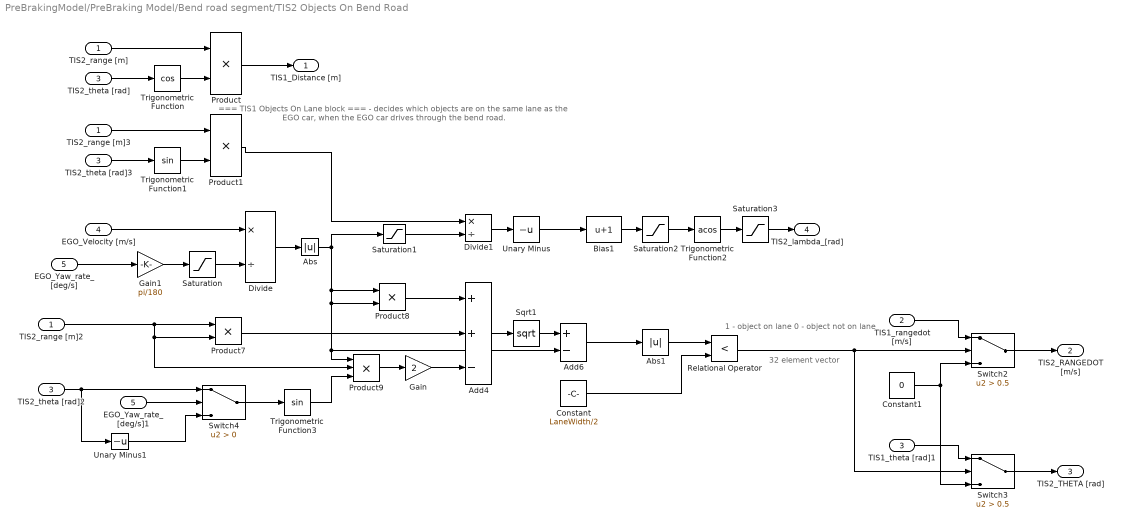
== system PreBrakingModel/PreBraking Model/Bend road segment/TIS2 Objects On Bend Road ==
  note: 1  - object      on lane
      | 0 - object not on lane
  note: 32 element vector
  note: === TIS1 Objects On Lane block ===
      |
      |  - decides which objects are on the same lane as the EGO car,
      |     when the EGO car drives through the bend road.
  TIS2_range [m] : Inport
  TIS1_rangedot [m/s] : Inport  Port=2
  TIS2_theta [rad] : Inport  Port=3
  EGO_Velocity [m/s] : Inport  Port=4
  EGO_Yaw_rate_[deg/s] : Inport  Port=5
  Abs : Abs
  Abs1 : Abs
  Add4 : Sum  Inputs=++-
  Add6 : Sum  Inputs=+-
  Bias1 : Bias  Bias=1
  Constant : Constant  Value=LaneWidth/2
  Constant1 : Constant  Value=0
  Divide : Product  Inputs=*/
  Divide1 : Product  Inputs=*/
  EGO_Yaw_rate_[deg/s]1 : InportShadow  Port=5
  Gain : Gain  Gain=2
  Gain1 : Gain  Gain=pi/180
  Product{,1,7..8} (4 alike) : Product  RndMeth=Zero
  Product9 : Product  Inputs=3  RndMeth=Zero
  Relational Operator : RelationalOperator  Operator=<  OutDataTypeStr=boolean
  Saturation : Saturate  UpperLimit=inf  LowerLimit=1e-6
  Saturation1 : Saturate  UpperLimit=inf  LowerLimit=1e-6
  Saturation2 : Saturate  UpperLimit=1  LowerLimit=-1
  Saturation3 : Saturate  UpperLimit=pi  LowerLimit=0
  Sqrt1 : Math  Operator=sqrt  SaturateOnIntegerOverflow=on
  Switch2 : Switch  Criteria=u2 > Threshold  Threshold=0.5
  Switch3 : Switch  Criteria=u2 > Threshold  Threshold=0.5
  Switch4 : Switch  Criteria=u2 > Threshold
  TIS1_theta [rad]1 : InportShadow  Port=3
  TIS2_range [m]2 : InportShadow
  TIS2_range [m]3 : InportShadow
  TIS2_theta [rad]2 : InportShadow  Port=3
  TIS2_theta [rad]3 : InportShadow  Port=3
  Trigonometric Function : Trigonometry  Operator=cos
  Trigonometric Function1 : Trigonometry
  Trigonometric Function2 : Trigonometry  Operator=acos
  Trigonometric Function3 : Trigonometry
  Unary Minus : UnaryMinus
  Unary Minus1 : UnaryMinus
  TIS1_Distance [m] : Outport
  TIS2_RANGEDOT [m/s] : Outport  Port=2
  TIS2_THETA [rad] : Outport  Port=3
  TIS2_lambda_[rad] : Outport  Port=4
  wires:
  TIS2_range [m]/1 -> Product/1
  TIS2_theta [rad]/1 -> Trigonometric Function/1
  Trigonometric Function/1 -> Product/2
  Trigonometric Function1/1 -> Product1/2
  EGO_Velocity [m/s]/1 -> Divide/1
  EGO_Yaw_rate_[deg/s]/1 -> Gain1/1
  Divide/1 -> Abs/1
  Relational Operator/1 -> Switch2/2, Switch3/2
  TIS1_rangedot [m/s]/1 -> Switch2/1
  TIS1_theta [rad]1/1 -> Switch3/1
  Constant1/1 -> Switch2/3, Switch3/3
  Switch2/1 -> TIS2_RANGEDOT [m/s]/1
  Switch3/1 -> TIS2_THETA [rad]/1
  Bias1/1 -> Saturation2/1
  Divide1/1 -> Unary Minus/1
  Unary Minus/1 -> Bias1/1
  Trigonometric Function2/1 -> Saturation3/1
  Abs/1 -> Product8/1, Product8/2, Product9/1, Add6/2, Saturation1/1
  Product/1 -> TIS1_Distance [m]/1
  Product8/1 -> Add4/1
  Product7/1 -> Add4/2
  Gain/1 -> Add4/3
  Product9/1 -> Gain/1
  Trigonometric Function3/1 -> Product9/3
  Add4/1 -> Sqrt1/1
  Sqrt1/1 -> Add6/1
  Add6/1 -> Abs1/1
  EGO_Yaw_rate_[deg/s]1/1 -> Switch4/2
  Switch4/1 -> Trigonometric Function3/1
  TIS2_theta [rad]2/1 -> Unary Minus1/1, Switch4/1
  TIS2_range [m]2/1 -> Product7/1, Product7/2, Product9/2
  TIS2_range [m]3/1 -> Product1/1
  TIS2_theta [rad]3/1 -> Trigonometric Function1/1
  Product1/1 -> Divide1/1
  Abs1/1 -> Relational Operator/1
  Constant/1 -> Relational Operator/2
  Saturation/1 -> Divide/2
  Saturation1/1 -> Divide1/2
  Saturation2/1 -> Trigonometric Function2/1
  Saturation3/1 -> TIS2_lambda_[rad]/1
  Gain1/1 -> Saturation/1
  Unary Minus1/1 -> Switch4/3

== system PreBrakingModel/PreBraking Model/Bend road segment/TIS2 TTC Computing1 ==
  Distance [m] : Inport
  Velocity [m/s] : Inport  Port=2
  Compare : simulink/Logic and Bit Operations/Compare To Constant  relop===  const=1e-6  OutDataTypeStr=uint8  ZeroCross=off
  Constant : Constant  Value=0
  Data Type Conversion : DataTypeConversion
  Product : Product  Inputs=*/  RndMeth=Zero
  Saturation : Saturate  UpperLimit=inf  LowerLimit=1e-6
  Switch : Switch  Criteria=u2 > Threshold
  Switch1 : Switch  Criteria=u2 > Threshold  Threshold=0.5
  TTC [s] : Outport
  wires:
  Velocity [m/s]/1 -> Switch/2, Switch/1
  Constant/1 -> Switch/3, Switch1/1
  Switch/1 -> Saturation/1
  Distance [m]/1 -> Product/1
  Saturation/1 -> Product/2, Compare/1
  Compare/1 -> Data Type Conversion/1
  Product/1 -> Switch1/3
  Switch1/1 -> TTC [s]/1
  Data Type Conversion/1 -> Switch1/2

== system PreBrakingModel/PreBraking Model/Braking Lights/If Action Subsystem ==
  In1 : Inport
  Action Port : ActionPort  PropagateVarSize=During execution  ActionType=then
  Add : Sum
  Constant : Constant
  Unary Minus : UnaryMinus
  left light : Outport
  right light : Outport  Port=2
  wires:
  In1/1 -> left light/1, Unary Minus/1
  Add/1 -> right light/1
  Unary Minus/1 -> Add/1
  Constant/1 -> Add/2
